simulink model "continous"  (R2018b)
settings: Solver=VariableStepAuto  StartTime=0.0  StopTime=10.0  RelTol=1e-3
undefined symbols (not defined in the file): a, Be, fc, Ke, Ki, Kp
settings Model: Creator=adam  LastModifiedBy=adam

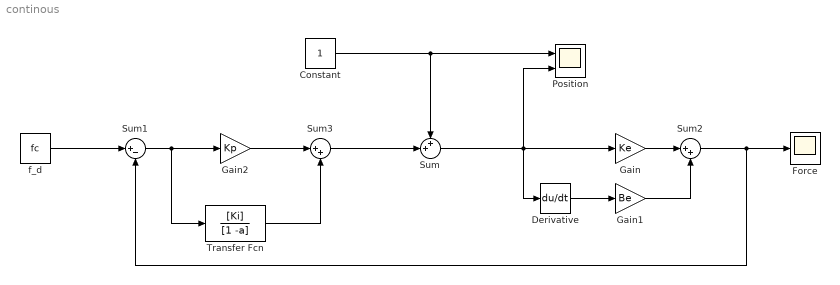
== system continous ==
  Constant : Constant
  Derivative : Derivative
  Force : Scope
  Gain : Gain  Gain=Ke
  Gain1 : Gain  Gain=Be
  Gain2 : Gain  Gain=Kp
  Position : Scope  NumInputPorts=2
  Sum : Sum  Inputs=++|
  Sum1 : Sum  Inputs=|+-
  Sum2 : Sum  Inputs=|++
  Sum3 : Sum  Inputs=|++
  Transfer Fcn : TransferFcn  Numerator=[Ki]  Denominator=[1 -a]
  f_d : Constant  Value=fc
  wires:
  Gain/1 -> Sum2/1
  Derivative/1 -> Gain1/1
  Sum/1 -> Position/2, Gain/1, Derivative/1
  Gain1/1 -> Sum2/2
  Transfer Fcn/1 -> Sum3/2
  Gain2/1 -> Sum3/1
  Sum1/1 -> Transfer Fcn/1, Gain2/1
  Sum3/1 -> Sum/2
  Sum2/1 -> Sum1/2, Force/1
  f_d/1 -> Sum1/1
  Constant/1 -> Sum/1, Position/1
